simulink model "Model_Simulation"  (R2016a)
settings: Solver=FixedStepAuto  StartTime=0.0  StopTime=5  FixedStep=2e-6  RelTol=1e-3
values from neighbouring files (symbols this model uses):
  C = 3060e-6    (= 0.00306)    [Controle_Inversor_UR_D.m]
  Ki_i_disc = wc*Rf    (= 44.2477838534)    [Controle_Inversor_UR_D.m]
  Ki_i_disc_b = wc_b*Rb/Vdc    (= 0.0983284085631)    [Controle_Inversor_UR_D.m]
  Ki_q_disc = wq/H    [Controle_Inversor_UR_D.m]
  Ki_v_disc_b = wc_bv/Req    (= 14.5799013102)    [Controle_Inversor_UR_D.m]
  Ki_vdc_disc = ((wvdc)^2*C)/Gt    [Controle_Inversor_UR_D.m]
  Kp_i_disc = wc*Lf    (= 2.19688771906)    [Controle_Inversor_UR_D.m]
  Kp_i_disc_b = wc_b*Lb/Vdc    (= 0.00545604673435)    [Controle_Inversor_UR_D.m]
  Kp_q_disc = Ki_q_disc*(Lf/Kp_i_disc)    [Controle_Inversor_UR_D.m]
  Kp_v_disc_b = wc_bv*Cin    (= 0.0356301510224)    [Controle_Inversor_UR_D.m]
  Kp_vdc_disc = (2*ksi_vdc*wvdc*C)/Gt    [Controle_Inversor_UR_D.m]
  Lf = (0.0012+2.8949e-04)    (= 0.00148949)    [Controle_Inversor_UR_D.m]
  Tsw = 1/fsw    (= 0.0002)    [Controle_Inversor_UR_D.m]
  w = 2*pi*60    (= 376.991118431)    [Controle_Inversor_UR_D.m]
undefined symbols (not defined in the file or in its folder): D1, dEgdT, Delta, EgRef, gcbh, k1, Rsh_array5pc, sigbuilder_block, sps_rtmsupport, Tref_K, VT_ref
libraries: powerlib x179, simulink x14, powerlib_meascontrol x13, spsPVarrayModel x12
(part 1 of 20)
settings Model: Creator=lucca  LastModifiedBy=lucca

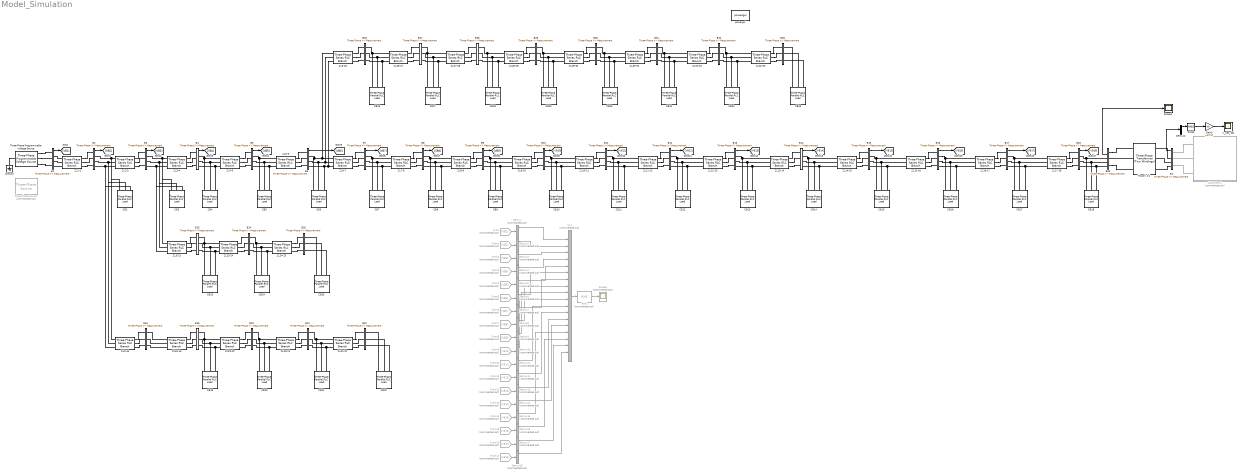
== system Model_Simulation ==
  B1 : powerlib/Measurements/Three-Phase V-I Measurement  VoltageMeasurement=phase-to-ground  SetLabelV=off  LabelV=Vabc  Vpu=off  VpuLL=off  CurrentMeasurement=yes  SetLabelI=off  LabelI=Iabc  Ipu=off  Pbase=100e6  Vbase=1.06  OutputType=Complex  PhasorSimulation=off  PSBequivalent=0
  "B1 " : powerlib/Measurements/Three-Phase V-I Measurement  VoltageMeasurement=phase-to-phase  SetLabelV=off  LabelV=Vabc  Vpu=off  VpuLL=off  CurrentMeasurement=no  SetLabelI=off  LabelI=Iabc  Ipu=off  Pbase=100e6  Vbase=1.06  OutputType=Complex  PhasorSimulation=off  PSBequivalent=0
  B{2..18} (17 alike) : powerlib/Measurements/Three-Phase V-I Measurement  VoltageMeasurement=phase-to-phase  SetLabelV=off  LabelV=Vabc  Vpu=off  VpuLL=off  CurrentMeasurement=no  SetLabelI=off  LabelI=Iabc  Ipu=off  Pbase=100e6  Vbase=1.06  OutputType=Complex  PhasorSimulation=off  PSBequivalent=0
  B{19..34} (16 alike) : powerlib/Measurements/Three-Phase V-I Measurement  VoltageMeasurement=no  SetLabelV=off  LabelV=Vabc  Vpu=off  VpuLL=off  CurrentMeasurement=no  SetLabelI=off  LabelI=Iabc  Ipu=off  Pbase=100e6  Vbase=1.06  OutputType=Complex  PhasorSimulation=off  PSBequivalent=0
  B35 : powerlib/Measurements/Three-Phase V-I Measurement  VoltageMeasurement=phase-to-ground  SetLabelV=off  LabelV=Vabc  Vpu=off  VpuLL=off  CurrentMeasurement=yes  SetLabelI=off  LabelI=Iabc  Ipu=off  Pbase=100e6  Vbase=1.06  OutputType=Complex  PhasorSimulation=off  PSBequivalent=0
  CB{6,9..10,16..17,28} (6 alike) : powerlib/Elements/Three-Phase Parallel RLC Load  LConnTagsString=A|B|C  Configuration=Y (grounded)  NominalVoltage=13.8e3  Vabc=[1e3 1e3 1e3]  Vabcp=[1e3 1e3 1e3]  NominalFrequency=60  UnbalancedPower=off  ActivePower=0.06e6  InductivePower=0.02e6  CapacitivePower=0  Pabc=[10e3 9e3 11e3]  QLabc=[100 90 110]  QCabc=[100 90 110]  Pabcp=[10e3 9e3 11e3]  QLabcp=[100 90 110]  QCabcp=[100 90 110]  Measurements=None  LoadType=constant Z
  CB11 : powerlib/Elements/Three-Phase Parallel RLC Load  LConnTagsString=A|B|C  Configuration=Y (grounded)  NominalVoltage=13.8e3  Vabc=[1e3 1e3 1e3]  Vabcp=[1e3 1e3 1e3]  NominalFrequency=60  UnbalancedPower=off  ActivePower=0.045e6  InductivePower=0.03e6  CapacitivePower=0  Pabc=[10e3 9e3 11e3]  QLabc=[100 90 110]  QCabc=[100 90 110]  Pabcp=[10e3 9e3 11e3]  QLabcp=[100 90 110]  QCabcp=[100 90 110]  Measurements=None  LoadType=constant Z
  CB12 : powerlib/Elements/Three-Phase Parallel RLC Load  LConnTagsString=A|B|C  Configuration=Y (grounded)  NominalVoltage=13.8e3  Vabc=[1e3 1e3 1e3]  Vabcp=[1e3 1e3 1e3]  NominalFrequency=60  UnbalancedPower=off  ActivePower=0.06e6  InductivePower=0.035e6  CapacitivePower=0  Pabc=[10e3 9e3 11e3]  QLabc=[100 90 110]  QCabc=[100 90 110]  Pabcp=[10e3 9e3 11e3]  QLabcp=[100 90 110]  QCabcp=[100 90 110]  Measurements=None  LoadType=constant Z
  CB13 : powerlib/Elements/Three-Phase Parallel RLC Load  LConnTagsString=A|B|C  Configuration=Y (grounded)  NominalVoltage=13.8e3  Vabc=[1e3 1e3 1e3]  Vabcp=[1e3 1e3 1e3]  NominalFrequency=60  UnbalancedPower=off  ActivePower=0.06e6  InductivePower=0.035e6  CapacitivePower=0  Pabc=[10e3 9e3 11e3]  QLabc=[100 90 110]  QCabc=[100 90 110]  Pabcp=[10e3 9e3 11e3]  QLabcp=[100 90 110]  QCabcp=[100 90 110]  Measurements=None  LoadType=constant Z
  CB14 : powerlib/Elements/Three-Phase Parallel RLC Load  LConnTagsString=A|B|C  Configuration=Y (grounded)  NominalVoltage=13.8e3  Vabc=[1e3 1e3 1e3]  Vabcp=[1e3 1e3 1e3]  NominalFrequency=60  UnbalancedPower=off  ActivePower=0.12e6  InductivePower=0.08e6  CapacitivePower=0  Pabc=[10e3 9e3 11e3]  QLabc=[100 90 110]  QCabc=[100 90 110]  Pabcp=[10e3 9e3 11e3]  QLabcp=[100 90 110]  QCabcp=[100 90 110]  Measurements=None  LoadType=constant Z
  CB15 : powerlib/Elements/Three-Phase Parallel RLC Load  LConnTagsString=A|B|C  Configuration=Y (grounded)  NominalVoltage=13.8e3  Vabc=[1e3 1e3 1e3]  Vabcp=[1e3 1e3 1e3]  NominalFrequency=60  UnbalancedPower=off  ActivePower=0.06e6  InductivePower=0.01e6  CapacitivePower=0  Pabc=[10e3 9e3 11e3]  QLabc=[100 90 110]  QCabc=[100 90 110]  Pabcp=[10e3 9e3 11e3]  QLabcp=[100 90 110]  QCabcp=[100 90 110]  Measurements=None  LoadType=constant Z
  CB{3,18..22} (6 alike) : powerlib/Elements/Three-Phase Parallel RLC Load  LConnTagsString=A|B|C  Configuration=Y (grounded)  NominalVoltage=13.8e3  Vabc=[1e3 1e3 1e3]  Vabcp=[1e3 1e3 1e3]  NominalFrequency=60  UnbalancedPower=off  ActivePower=0.09e6  InductivePower=0.04e6  CapacitivePower=0  Pabc=[10e3 9e3 11e3]  QLabc=[100 90 110]  QCabc=[100 90 110]  Pabcp=[10e3 9e3 11e3]  QLabcp=[100 90 110]  QCabcp=[100 90 110]  Measurements=None  LoadType=constant Z
  CB2 : powerlib/Elements/Three-Phase Parallel RLC Load  LConnTagsString=A|B|C  Configuration=Y (grounded)  NominalVoltage=13.8e3  Vabc=[1e3 1e3 1e3]  Vabcp=[1e3 1e3 1e3]  NominalFrequency=60  UnbalancedPower=off  ActivePower=0.1e6  InductivePower=0.06e6  CapacitivePower=0  Pabc=[10e3 9e3 11e3]  QLabc=[100 90 110]  QCabc=[100 90 110]  Pabcp=[10e3 9e3 11e3]  QLabcp=[100 90 110]  QCabcp=[100 90 110]  Measurements=None  LoadType=constant Z
  CB23 : powerlib/Elements/Three-Phase Parallel RLC Load  LConnTagsString=A|B|C  Configuration=Y (grounded)  NominalVoltage=13.8e3  Vabc=[1e3 1e3 1e3]  Vabcp=[1e3 1e3 1e3]  NominalFrequency=60  UnbalancedPower=off  ActivePower=0.09e6  InductivePower=0.05e6  CapacitivePower=0  Pabc=[10e3 9e3 11e3]  QLabc=[100 90 110]  QCabc=[100 90 110]  Pabcp=[10e3 9e3 11e3]  QLabcp=[100 90 110]  QCabcp=[100 90 110]  Measurements=None  LoadType=constant Z
  CB24 : powerlib/Elements/Three-Phase Parallel RLC Load  LConnTagsString=A|B|C  Configuration=Y (grounded)  NominalVoltage=13.8e3  Vabc=[1e3 1e3 1e3]  Vabcp=[1e3 1e3 1e3]  NominalFrequency=60  UnbalancedPower=off  ActivePower=0.42e6  InductivePower=0.2e6  CapacitivePower=0  Pabc=[10e3 9e3 11e3]  QLabc=[100 90 110]  QCabc=[100 90 110]  Pabcp=[10e3 9e3 11e3]  QLabcp=[100 90 110]  QCabcp=[100 90 110]  Measurements=None  LoadType=constant Z
  CB25 : powerlib/Elements/Three-Phase Parallel RLC Load  LConnTagsString=A|B|C  Configuration=Y (grounded)  NominalVoltage=13.8e3  Vabc=[1e3 1e3 1e3]  Vabcp=[1e3 1e3 1e3]  NominalFrequency=60  UnbalancedPower=off  ActivePower=0.42e6  InductivePower=0.2e6  CapacitivePower=0  Pabc=[10e3 9e3 11e3]  QLabc=[100 90 110]  QCabc=[100 90 110]  Pabcp=[10e3 9e3 11e3]  QLabcp=[100 90 110]  QCabcp=[100 90 110]  Measurements=None  LoadType=constant Z
  CB26 : powerlib/Elements/Three-Phase Parallel RLC Load  LConnTagsString=A|B|C  Configuration=Y (grounded)  NominalVoltage=13.8e3  Vabc=[1e3 1e3 1e3]  Vabcp=[1e3 1e3 1e3]  NominalFrequency=60  UnbalancedPower=off  ActivePower=0.06e6  InductivePower=0.025e6  CapacitivePower=0  Pabc=[10e3 9e3 11e3]  QLabc=[100 90 110]  QCabc=[100 90 110]  Pabcp=[10e3 9e3 11e3]  QLabcp=[100 90 110]  QCabcp=[100 90 110]  Measurements=None  LoadType=constant Z
  CB27 : powerlib/Elements/Three-Phase Parallel RLC Load  LConnTagsString=A|B|C  Configuration=Y (grounded)  NominalVoltage=13.8e3  Vabc=[1e3 1e3 1e3]  Vabcp=[1e3 1e3 1e3]  NominalFrequency=60  UnbalancedPower=off  ActivePower=0.06e6  InductivePower=0.025e6  CapacitivePower=0  Pabc=[10e3 9e3 11e3]  QLabc=[100 90 110]  QCabc=[100 90 110]  Pabcp=[10e3 9e3 11e3]  QLabcp=[100 90 110]  QCabcp=[100 90 110]  Measurements=None  LoadType=constant Z
  CB29 : powerlib/Elements/Three-Phase Parallel RLC Load  LConnTagsString=A|B|C  Configuration=Y (grounded)  NominalVoltage=13.8e3  Vabc=[1e3 1e3 1e3]  Vabcp=[1e3 1e3 1e3]  NominalFrequency=60  UnbalancedPower=off  ActivePower=0.12e6  InductivePower=0.07e6  CapacitivePower=0  Pabc=[10e3 9e3 11e3]  QLabc=[100 90 110]  QCabc=[100 90 110]  Pabcp=[10e3 9e3 11e3]  QLabcp=[100 90 110]  QCabcp=[100 90 110]  Measurements=None  LoadType=constant Z
  CB30 : powerlib/Elements/Three-Phase Parallel RLC Load  LConnTagsString=A|B|C  Configuration=Y (grounded)  NominalVoltage=13.8e3  Vabc=[1e3 1e3 1e3]  Vabcp=[1e3 1e3 1e3]  NominalFrequency=60  UnbalancedPower=off  ActivePower=0.2e6  InductivePower=0.1e6  CapacitivePower=0  Pabc=[10e3 9e3 11e3]  QLabc=[100 90 110]  QCabc=[100 90 110]  Pabcp=[10e3 9e3 11e3]  QLabcp=[100 90 110]  QCabcp=[100 90 110]  Measurements=None  LoadType=constant Z
  CB31 : powerlib/Elements/Three-Phase Parallel RLC Load  LConnTagsString=A|B|C  Configuration=Y (grounded)  NominalVoltage=13.8e3  Vabc=[1e3 1e3 1e3]  Vabcp=[1e3 1e3 1e3]  NominalFrequency=60  UnbalancedPower=off  ActivePower=0.15e6  InductivePower=0.07e6  CapacitivePower=0  Pabc=[10e3 9e3 11e3]  QLabc=[100 90 110]  QCabc=[100 90 110]  Pabcp=[10e3 9e3 11e3]  QLabcp=[100 90 110]  QCabcp=[100 90 110]  Measurements=None  LoadType=constant Z
  CB32 : powerlib/Elements/Three-Phase Parallel RLC Load  LConnTagsString=A|B|C  Configuration=Y (grounded)  NominalVoltage=13.8e3  Vabc=[1e3 1e3 1e3]  Vabcp=[1e3 1e3 1e3]  NominalFrequency=60  UnbalancedPower=off  ActivePower=0.21e6  InductivePower=0.1e6  CapacitivePower=0  Pabc=[10e3 9e3 11e3]  QLabc=[100 90 110]  QCabc=[100 90 110]  Pabcp=[10e3 9e3 11e3]  QLabcp=[100 90 110]  QCabcp=[100 90 110]  Measurements=None  LoadType=constant Z
  CB33 : powerlib/Elements/Three-Phase Parallel RLC Load  LConnTagsString=A|B|C  Configuration=Y (grounded)  NominalVoltage=13.8e3  Vabc=[1e3 1e3 1e3]  Vabcp=[1e3 1e3 1e3]  NominalFrequency=60  UnbalancedPower=off  ActivePower=0.06e6  InductivePower=0.04e6  CapacitivePower=0  Pabc=[10e3 9e3 11e3]  QLabc=[100 90 110]  QCabc=[100 90 110]  Pabcp=[10e3 9e3 11e3]  QLabcp=[100 90 110]  QCabcp=[100 90 110]  Measurements=None  LoadType=constant Z
  CB4 : powerlib/Elements/Three-Phase Parallel RLC Load  LConnTagsString=A|B|C  Configuration=Y (grounded)  NominalVoltage=13.8e3  Vabc=[1e3 1e3 1e3]  Vabcp=[1e3 1e3 1e3]  NominalFrequency=60  UnbalancedPower=off  ActivePower=0.12e6  InductivePower=0.08e6  CapacitivePower=0  Pabc=[10e3 9e3 11e3]  QLabc=[100 90 110]  QCabc=[100 90 110]  Pabcp=[10e3 9e3 11e3]  QLabcp=[100 90 110]  QCabcp=[100 90 110]  Measurements=None  LoadType=constant Z
  CB5 : powerlib/Elements/Three-Phase Parallel RLC Load  LConnTagsString=A|B|C  Configuration=Y (grounded)  NominalVoltage=13.8e3  Vabc=[1e3 1e3 1e3]  Vabcp=[1e3 1e3 1e3]  NominalFrequency=60  UnbalancedPower=off  ActivePower=0.06e6  InductivePower=0.03e6  CapacitivePower=0  Pabc=[10e3 9e3 11e3]  QLabc=[100 90 110]  QCabc=[100 90 110]  Pabcp=[10e3 9e3 11e3]  QLabcp=[100 90 110]  QCabcp=[100 90 110]  Measurements=None  LoadType=constant Z
  CB7 : powerlib/Elements/Three-Phase Parallel RLC Load  LConnTagsString=A|B|C  Configuration=Y (grounded)  NominalVoltage=13.8e3  Vabc=[1e3 1e3 1e3]  Vabcp=[1e3 1e3 1e3]  NominalFrequency=60  UnbalancedPower=off  ActivePower=0.2e6  InductivePower=0.1e6  CapacitivePower=0  Pabc=[10e3 9e3 11e3]  QLabc=[100 90 110]  QCabc=[100 90 110]  Pabcp=[10e3 9e3 11e3]  QLabcp=[100 90 110]  QCabcp=[100 90 110]  Measurements=None  LoadType=constant Z
  CB8 : powerlib/Elements/Three-Phase Parallel RLC Load  LConnTagsString=A|B|C  Configuration=Y (grounded)  NominalVoltage=13.8e3  Vabc=[1e3 1e3 1e3]  Vabcp=[1e3 1e3 1e3]  NominalFrequency=60  UnbalancedPower=off  ActivePower=0.2e6  InductivePower=0.1e6  CapacitivePower=0  Pabc=[10e3 9e3 11e3]  QLabc=[100 90 110]  QCabc=[100 90 110]  Pabcp=[10e3 9e3 11e3]  QLabcp=[100 90 110]  QCabcp=[100 90 110]  Measurements=None  LoadType=constant Z
  Demux{,1,3..18} (18 alike) : Demux  Commented=on  Outputs=3
  Demux2 : Demux  Outputs=3
  From : From  Commented=on  GotoTag=VB1
  From1 : From  Commented=on  GotoTag=VB2
  From10 : From  Commented=on  GotoTag=VB11
  From11 : From  Commented=on  GotoTag=VB12
  From12 : From  Commented=on  GotoTag=VB13
  From13 : From  Commented=on  GotoTag=VB14
  From14 : From  Commented=on  GotoTag=VB15
  From15 : From  Commented=on  GotoTag=VB16
  From16 : From  Commented=on  GotoTag=VB17
  From17 : From  Commented=on  GotoTag=VB18
  From2 : From  Commented=on  GotoTag=VB3
  From3 : From  Commented=on  GotoTag=VB4
  From4 : From  Commented=on  GotoTag=VB5
  From5 : From  Commented=on  GotoTag=VB6
  From6 : From  Commented=on  GotoTag=VB7
  From7 : From  Commented=on  GotoTag=VB8
  From8 : From  Commented=on  GotoTag=VB9
  From9 : From  Commented=on  GotoTag=VB10
  Gain3 : Gain  Gain=sqrt(2)
  Ground : powerlib/Elements/Ground  LConnTagsString=a
  Mux : Mux  Commented=on  Inputs=18
  RMS : powerlib_meascontrol/Measurements/RMS  Commented=on  TrueRMS=on  Freq=60  RMSInit=13800  Ts=0
  RMS5 : powerlib_meascontrol/Measurements/RMS  TrueRMS=on  Freq=60  RMSInit=120  Ts=0
  Scope2 : Scope
  Scope3 : Scope  Commented=on
  Subsystem2 : Subsystem  Commented=on
  Three-Phase Programmable Voltage Source : powerlib/Electrical Sources/Three-Phase Programmable Voltage Source  PositiveSequence=[13.8e3 0 60]  VariationEntity=Amplitude  VariationType=Table of time-amplitude pairs  VariationTypeAlt=Step  VariationStep=0.5  VariationRate=10  VariationMagnitude=0.3  VariationFrequency=2  VariationTiming=[1 2]  VariationPhaseA=off  Amplitudes=[1 0.7 1]  TimeValues=[0 2 3]  HarmonicGeneration=off  HarmonicA=[3 0.2 -25 0]  HarmonicB=[2 0.15 35 2]  Timing="[0.05  3]"  BusType=swing  Pref=0  Qref=0  Qmin=-inf  Qmax=inf
  Three-Phase Source : powerlib/Electrical Sources/Three-Phase Source  Commented=on  InternalConnection=Yg  VoltagePhases=off  Voltage=13.8e3  PhaseAngle=0  Voltage_phases=[25e3 25e3 25e3]/sqrt(3)  PhaseAngles_phases=[0 -120 +120]  Frequency=60  NonIdealSource=off  SpecifyImpedance=off  Resistance=0.8929  Inductance=16.58e-3  ShortCircuitLevel=100e6  BaseVoltage=25e3  XRratio=7  BusType=swing  Pref=10e3  Qref=0  Prefabc=[10e3, 10e3, 10e3]  Qrefabc=[0, 0, 0]  Qmin=-inf  Qmax=inf
  Transf. 4-1 : powerlib/Elements/Three-Phase Transformer (Two Windings)  Winding1Connection=Delta (D1)  Winding2Connection=Yg  CoreType=Three single-phase transformers  SetSaturation=off  Hysteresis=off  DataFile='hysteresis'  SetInitialFlux=off  Measurements=None  UNITS=pu  NominalPower=[ 300e3 , 60 ]  Winding1=[13800 0 0.05/2]  Winding2=[800 0 0.05/2]  Rm=370.3704  Lm=14.4834  L0=0.49999  Saturation=[0 0;0.006 1.2;2.4999 1.52]  InitialFluxes=[0.80003 -0.80003 0.70001]  MoreParameters=off  BreakLoop=off  DataType=off  TransfoNumber=1
  V_sec_GD : Scope
  ZL1-2 : powerlib/Elements/Three-Phase Series RLC Branch  LConnTagsString=A|B|C  RConnTagsString=A|B|C  BranchType=RL  Resistance=0.057525912  Inductance=7.7784e-05  Capacitance=1e-6  Measurements=None
  ZL10-11 : powerlib/Elements/Three-Phase Series RLC Branch  LConnTagsString=A|B|C  RConnTagsString=A|B|C  BranchType=RL  Resistance=0.122663712  Inductance=1.0758e-04  Capacitance=1e-6  Measurements=None
  ZL11-12 : powerlib/Elements/Three-Phase Series RLC Branch  LConnTagsString=A|B|C  RConnTagsString=A|B|C  BranchType=RL  Resistance=0.233597628  Inductance=2.0489e-04  Capacitance=1e-6  Measurements=None
  ZL12-13 : powerlib/Elements/Three-Phase Series RLC Branch  LConnTagsString=A|B|C  RConnTagsString=A|B|C  BranchType=RL  Resistance=0.915922324  Inductance=0.0019  Capacitance=1e-6  Measurements=None
  ZL13-14 : powerlib/Elements/Three-Phase Series RLC Branch  LConnTagsString=A|B|C  RConnTagsString=A|B|C  BranchType=RL  Resistance=0.337917936  Inductance=0.0012  Capacitance=1e-6  Measurements=None
  ZL14-15 : powerlib/Elements/Three-Phase Series RLC Branch  LConnTagsString=A|B|C  RConnTagsString=A|B|C  BranchType=RL  Resistance=0.368739846  Inductance=8.7054e-04  Capacitance=1e-6  Measurements=None
  ZL15-16 : powerlib/Elements/Three-Phase Series RLC Branch  LConnTagsString=A|B|C  RConnTagsString=A|B|C  BranchType=RL  Resistance=0.465635443  Inductance=9.0198e-04  Capacitance=1e-6  Measurements=None
  ZL16-17 : powerlib/Elements/Three-Phase Series RLC Branch  LConnTagsString=A|B|C  RConnTagsString=A|B|C  BranchType=RL  Resistance=0.804239697  Inductance=0.0028  Capacitance=1e-6  Measurements=None
  ZL17-18 : powerlib/Elements/Three-Phase Series RLC Branch  LConnTagsString=A|B|C  RConnTagsString=A|B|C  BranchType=RL  Resistance=0.456713311  Inductance=9.4998e-04  Capacitance=1e-6  Measurements=None
  ZL19-20 : powerlib/Elements/Three-Phase Series RLC Branch  LConnTagsString=A|B|C  RConnTagsString=A|B|C  BranchType=RL  Resistance=0.938508419  Inductance=0.0022  Capacitance=1e-6  Measurements=None
  ZL2-3 : powerlib/Elements/Three-Phase Series RLC Branch  LConnTagsString=A|B|C  RConnTagsString=A|B|C  BranchType=RL  Resistance=0.307595167  Inductance=4.1557e-04  Capacitance=1e-6  Measurements=None
  ZL2-34 : powerlib/Elements/Three-Phase Series RLC Branch  LConnTagsString=A|B|C  RConnTagsString=A|B|C  BranchType=RL  Resistance=0.057525912  Inductance=7.7784e-05  Capacitance=1e-6  Measurements=None
  ZL20-21 : powerlib/Elements/Three-Phase Series RLC Branch  LConnTagsString=A|B|C  RConnTagsString=A|B|C  BranchType=RL  Resistance=0.255497406  Inductance=7.9176e-04  Capacitance=1e-6  Measurements=None
  ZL21-22 : powerlib/Elements/Three-Phase Series RLC Branch  LConnTagsString=A|B|C  RConnTagsString=A|B|C  BranchType=RL  Resistance=0.442300637  Inductance=0.0016  Capacitance=1e-6  Measurements=None
  ZL23-24 : powerlib/Elements/Three-Phase Series RLC Branch  LConnTagsString=A|B|C  RConnTagsString=A|B|C  BranchType=RL  Resistance=0.560284909  Inductance=0.0012  Capacitance=1e-6  Measurements=None
  ZL24-25 : powerlib/Elements/Three-Phase Series RLC Branch  LConnTagsString=A|B|C  RConnTagsString=A|B|C  BranchType=RL  Resistance=0.559037059  Inductance=0.0012  Capacitance=1e-6  Measurements=None
  ZL26-27 : powerlib/Elements/Three-Phase Series RLC Branch  LConnTagsString=A|B|C  RConnTagsString=A|B|C  BranchType=RL  Resistance=0.177319567  Inductance=2.3948e-04  Capacitance=1e-6  Measurements=None
  ZL27-28 : powerlib/Elements/Three-Phase Series RLC Branch  LConnTagsString=A|B|C  RConnTagsString=A|B|C  BranchType=RL  Resistance=0.660736881  Inductance=0.0015  Capacitance=1e-6  Measurements=None
  ZL28-29 : powerlib/Elements/Three-Phase Series RLC Branch  LConnTagsString=A|B|C  RConnTagsString=A|B|C  BranchType=RL  Resistance=0.501760717  Inductance=0.0012  Capacitance=1e-6  Measurements=None
  ZL29-30 : powerlib/Elements/Three-Phase Series RLC Branch  LConnTagsString=A|B|C  RConnTagsString=A|B|C  BranchType=RL  Resistance=0.316642084  Inductance=4.2782e-04  Capacitance=1e-6  Measurements=None
  ZL3-23 : powerlib/Elements/Three-Phase Series RLC Branch  LConnTagsString=A|B|C  RConnTagsString=A|B|C  BranchType=RL  Resistance=0.28151509  Inductance=5.1024e-04  Capacitance=1e-6  Measurements=None
  ZL3-4 : powerlib/Elements/Three-Phase Series RLC Branch  LConnTagsString=A|B|C  RConnTagsString=A|B|C  BranchType=RL  Resistance=0.228356656  Inductance=3.0850e-04  Capacitance=1e-6  Measurements=None
  ZL30-31 : powerlib/Elements/Three-Phase Series RLC Branch  LConnTagsString=A|B|C  RConnTagsString=A|B|C  BranchType=RL  Resistance=0.607952801  Inductance=0.0016  Capacitance=1e-6  Measurements=None
  ZL31-32 : powerlib/Elements/Three-Phase Series RLC Branch  LConnTagsString=A|B|C  RConnTagsString=A|B|C  BranchType=RL  Resistance=0.193728802  Inductance=5.9895e-04  Capacitance=1e-6  Measurements=None
  ZL32-33 : powerlib/Elements/Three-Phase Series RLC Branch  LConnTagsString=A|B|C  RConnTagsString=A|B|C  BranchType=RL  Resistance=0.212758523  Inductance=8.7749e-04  Capacitance=1e-6  Measurements=None
  ZL34-19 : powerlib/Elements/Three-Phase Series RLC Branch  LConnTagsString=A|B|C  RConnTagsString=A|B|C  BranchType=RL  Resistance=0.938508419  Inductance=0.0022  Capacitance=1e-6  Measurements=None
  ZL4-5 : powerlib/Elements/Three-Phase Series RLC Branch  LConnTagsString=A|B|C  RConnTagsString=A|B|C  BranchType=RL  Resistance=0.237777928  Inductance=3.2124e-04  Capacitance=1e-6  Measurements=None
  ZL5-6 : powerlib/Elements/Three-Phase Series RLC Branch  LConnTagsString=A|B|C  RConnTagsString=A|B|C  BranchType=RL  Resistance=0.510994811  Inductance=0.0012  Capacitance=1e-6  Measurements=None
  ZL6-26 : powerlib/Elements/Three-Phase Series RLC Branch  LConnTagsString=A|B|C  RConnTagsString=A|B|C  BranchType=RL  Resistance=0.126656834  Inductance=1.7113e-04  Capacitance=1e-6  Measurements=None
  ZL6-7 : powerlib/Elements/Three-Phase Series RLC Branch  LConnTagsString=A|B|C  RConnTagsString=A|B|C  BranchType=RL  Resistance=0.116798814  Inductance=0.0010  Capacitance=1e-6  Measurements=None
  ZL7-8 : powerlib/Elements/Three-Phase Series RLC Branch  LConnTagsString=A|B|C  RConnTagsString=A|B|C  BranchType=RL  Resistance=0.44386045  Inductance=3.8909e-04  Capacitance=1e-6  Measurements=None
  ZL8-9 : powerlib/Elements/Three-Phase Series RLC Branch  LConnTagsString=A|B|C  RConnTagsString=A|B|C  BranchType=RL  Resistance=0.642643047  Inductance=0.0012  Capacitance=1e-6  Measurements=None
  ZL9-10 : powerlib/Elements/Three-Phase Series RLC Branch  LConnTagsString=A|B|C  RConnTagsString=A|B|C  BranchType=RL  Resistance=0.651378001  Inductance=0.0012  Capacitance=1e-6  Measurements=None
  powergui : powerlib/powergui  Priority=1  SimulationMode=Discrete  SolverType=Tustin  SampleTime=2e-6  frequency=60  SPID=off  DisableSnubberDevices=off  DisableRonSwitches=off  DisableVfSwitches=off  SwTol=0  DisplayEquations=off  Interpol=off  ExternalGateDelay=off  methode=off  Ts=10  FunctionMessages=off  echomessages=off  HookPort=off  EnableUseOfTLC=off  x0status=blocks  frequencyindice=60  Pbase=100e6  ErrMax=0.0001  Iterations=50  UnitsV=kV  UnitsW=MW  buscounter=0  RestoreLinks=warning  ResistiveCurrentMeasurement=off  Frange=[0:2:500]  Ylog=off  Xlog=on  ShowGrid=off  save=off  variable=ZData  structure=0  ZoomFFT=off  StartTime=0.0  cycles=1  DisplayStyle=1  fundamental=60  FreqAxis=off  MaxFrequency=1000  frequencyindicesteady=1  RmsSteady=1  display=off
  wires:
  B1/1 -> Demux2/1
  RMS5/1 -> Gain3/1
  Gain3/1 -> V_sec_GD/1
  Demux2/1 -> RMS5/1
  "B1 "/1 -> [VB1]
  B2/1 -> [VB2]
  B3/1 -> [VB3]
  B4/1 -> [VB4]
  B5/1 -> [VB5]
  B6/1 -> [VB6]
  B7/1 -> [VB7]
  B8/1 -> [VB8]
  B9/1 -> [VB9]
  B10/1 -> [VB10]
  B11/1 -> [VB11]
  B12/1 -> [VB12]
  B13/1 -> [VB13]
  B14/1 -> [VB14]
  B15/1 -> [VB15]
  B16/1 -> [VB16]
  B17/1 -> [VB17]
  B18/1 -> [VB18]
  Mux/1 -> RMS/1
  Demux/1 -> Mux/1
  Demux1/1 -> Mux/2
  Demux3/1 -> Mux/3
  Demux4/1 -> Mux/4
  Demux5/1 -> Mux/5
  Demux6/1 -> Mux/6
  Demux7/1 -> Mux/7
  Demux8/1 -> Mux/8
  Demux9/1 -> Mux/9
  Demux10/1 -> Mux/10
  Demux11/1 -> Mux/11
  Demux12/1 -> Mux/12
  Demux13/1 -> Mux/13
  Demux14/1 -> Mux/14
  Demux15/1 -> Mux/15
  Demux16/1 -> Mux/16
  Demux17/1 -> Mux/17
  Demux18/1 -> Mux/18
  From/1 -> Demux/1
  From1/1 -> Demux1/1
  From2/1 -> Demux3/1
  From3/1 -> Demux4/1
  From4/1 -> Demux5/1
  From5/1 -> Demux6/1
  From6/1 -> Demux7/1
  From7/1 -> Demux8/1
  From8/1 -> Demux9/1
  From9/1 -> Demux10/1
  From10/1 -> Demux11/1
  From11/1 -> Demux12/1
  From12/1 -> Demux13/1
  From13/1 -> Demux14/1
  From14/1 -> Demux15/1
  From15/1 -> Demux16/1
  From16/1 -> Demux17/1
  From17/1 -> Demux18/1
  RMS/1 -> Scope3/1
  B35/2 -> Scope2/1
  connections:
  ZL1-2/LConn1 -- "B1 "/RConn1
  ZL1-2/LConn2 -- "B1 "/RConn2
  ZL1-2/LConn3 -- "B1 "/RConn3
  ZL1-2/RConn2 -- B2/LConn2
  ZL1-2/RConn1 -- B2/LConn1
  ZL1-2/RConn3 -- B2/LConn3
  ZL2-3/LConn1 -- ZL2-34/LConn1 -- CB2/LConn1 -- B2/RConn1
  ZL2-3/LConn2 -- ZL2-34/LConn2 -- CB2/LConn2 -- B2/RConn2
  ZL2-3/LConn3 -- CB2/LConn3 -- ZL2-34/LConn3 -- B2/RConn3
  ZL2-3/RConn3 -- B3/LConn3
  ZL2-3/RConn2 -- B3/LConn2
  ZL2-3/RConn1 -- B3/LConn1
  ZL3-4/LConn1 -- CB3/LConn1 -- ZL3-23/LConn1 -- B3/RConn1
  ZL3-4/LConn2 -- CB3/LConn2 -- ZL3-23/LConn2 -- B3/RConn2
  ZL3-4/LConn3 -- CB3/LConn3 -- ZL3-23/LConn3 -- B3/RConn3
  ZL3-4/RConn3 -- B4/LConn3
  ZL3-4/RConn2 -- B4/LConn2
  ZL3-4/RConn1 -- B4/LConn1
  ZL4-5/LConn1 -- CB4/LConn1 -- B4/RConn1
  ZL4-5/LConn2 -- CB4/LConn2 -- B4/RConn2
  ZL4-5/LConn3 -- B4/RConn3 -- CB4/LConn3
  B5/LConn3 -- ZL4-5/RConn3
  ZL4-5/RConn2 -- B5/LConn2
  ZL4-5/RConn1 -- B5/LConn1
  ZL5-6/LConn3 -- CB5/LConn3 -- B5/RConn3
  ZL5-6/LConn1 -- CB5/LConn1 -- B5/RConn1
  ZL5-6/RConn2 -- B6/LConn2
  ZL5-6/RConn1 -- B6/LConn1
  ZL5-6/LConn2 -- CB5/LConn2 -- B5/RConn2
  ZL5-6/RConn3 -- B6/LConn3
  ZL6-7/RConn2 -- B7/LConn2
  ZL6-7/LConn2 -- ZL6-26/LConn2 -- CB6/LConn2 -- B6/RConn2
  ZL6-7/LConn1 -- ZL6-26/LConn1 -- CB6/LConn1 -- B6/RConn1
  ZL6-7/LConn3 -- ZL6-26/LConn3 -- CB6/LConn3 -- B6/RConn3
  ZL6-7/RConn1 -- B7/LConn1
  ZL6-7/RConn3 -- B7/LConn3
  ZL7-8/RConn1 -- B8/LConn1
  ZL7-8/RConn3 -- B8/LConn3
  ZL7-8/LConn3 -- CB7/LConn3 -- B7/RConn3
  ZL7-8/RConn2 -- B8/LConn2
  ZL7-8/LConn2 -- CB7/LConn2 -- B7/RConn2
  ZL7-8/LConn1 -- CB7/LConn1 -- B7/RConn1
  ZL8-9/RConn3 -- B9/LConn3
  ZL8-9/LConn3 -- CB8/LConn3 -- B8/RConn3
  ZL8-9/RConn1 -- B9/LConn1
  ZL8-9/LConn2 -- CB8/LConn2 -- B8/RConn2
  ZL8-9/LConn1 -- CB8/LConn1 -- B8/RConn1
  ZL8-9/RConn2 -- B9/LConn2
  ZL9-10/LConn2 -- CB9/LConn2 -- B9/RConn2
  ZL9-10/RConn1 -- B10/LConn1
  ZL9-10/LConn1 -- CB9/LConn1 -- B9/RConn1
  ZL9-10/LConn3 -- CB9/LConn3 -- B9/RConn3
  ZL9-10/RConn2 -- B10/LConn2
  ZL9-10/RConn3 -- B10/LConn3
  ZL10-11/LConn1 -- B10/RConn1 -- CB10/LConn1
  ZL10-11/RConn2 -- B11/LConn2
  ZL10-11/RConn1 -- B11/LConn1
  ZL10-11/LConn3 -- CB10/LConn3 -- B10/RConn3
  ZL10-11/RConn3 -- B11/LConn3
  ZL10-11/LConn2 -- CB10/LConn2 -- B10/RConn2
  ZL11-12/LConn2 -- CB11/LConn2 -- B11/RConn2
  ZL11-12/LConn3 -- CB11/LConn3 -- B11/RConn3
  ZL11-12/RConn2 -- B12/LConn2
  ZL11-12/RConn1 -- B12/LConn1
  ZL11-12/RConn3 -- B12/LConn3
  ZL11-12/LConn1 -- CB11/LConn1 -- B11/RConn1
  ZL12-13/LConn2 -- CB12/LConn2 -- B12/RConn2
  ZL12-13/LConn3 -- CB12/LConn3 -- B12/RConn3
  ZL12-13/RConn2 -- B13/LConn2
  ZL12-13/LConn1 -- CB12/LConn1 -- B12/RConn1
  ZL12-13/RConn3 -- B13/LConn3
  ZL12-13/RConn1 -- B13/LConn1
  ZL13-14/RConn3 -- B14/LConn3
  ZL13-14/LConn1 -- CB13/LConn1 -- B13/RConn1
  ZL13-14/RConn1 -- B14/LConn1
  ZL13-14/RConn2 -- B14/LConn2
  ZL13-14/LConn3 -- CB13/LConn3 -- B13/RConn3
  ZL13-14/LConn2 -- CB13/LConn2 -- B13/RConn2
  ZL14-15/LConn1 -- CB14/LConn1 -- B14/RConn1
  ZL14-15/LConn3 -- CB14/LConn3 -- B14/RConn3
  ZL14-15/RConn2 -- B15/LConn2
  ZL14-15/RConn1 -- B15/LConn1
  ZL14-15/LConn2 -- CB14/LConn2 -- B14/RConn2
  ZL14-15/RConn3 -- B15/LConn3
  ZL15-16/RConn1 -- B16/LConn1
  ZL15-16/LConn3 -- CB15/LConn3 -- B15/RConn3
  ZL15-16/LConn1 -- CB15/LConn1 -- B15/RConn1
  ZL15-16/RConn3 -- B16/LConn3
  ZL15-16/RConn2 -- B16/LConn2
  ZL15-16/LConn2 -- CB15/LConn2 -- B15/RConn2
  B16/RConn2 -- CB16/LConn2 -- ZL16-17/LConn2
  ZL16-17/RConn2 -- B17/LConn2
  B16/RConn3 -- CB16/LConn3 -- ZL16-17/LConn3
  ZL16-17/RConn1 -- B17/LConn1
  ZL16-17/RConn3 -- B17/LConn3
  B16/RConn1 -- CB16/LConn1 -- ZL16-17/LConn1
  ZL17-18/LConn2 -- B17/RConn2 -- CB17/LConn2
  ZL17-18/LConn1 -- CB17/LConn1 -- B17/RConn1
  ZL17-18/LConn3 -- B17/RConn3 -- CB17/LConn3
  ZL17-18/RConn3 -- B18/LConn3
  ZL17-18/RConn1 -- B18/LConn1
  ZL17-18/RConn2 -- B18/LConn2
  ZL34-19/RConn2 -- B19/LConn2
  ZL2-34/RConn3 -- B34/LConn3
  ZL19-20/LConn3 -- CB19/LConn3 -- B19/RConn3
  ZL34-19/LConn1 -- B34/RConn1
  ZL20-21/RConn2 -- B21/LConn2
  ZL20-21/LConn2 -- B20/RConn2 -- CB20/LConn2
  ZL20-21/LConn1 -- CB20/LConn1 -- B20/RConn1
  ZL20-21/LConn3 -- CB20/LConn3 -- B20/RConn3
  ZL20-21/RConn1 -- B21/LConn1
  ZL20-21/RConn3 -- B21/LConn3
  ZL34-19/RConn1 -- B19/LConn1
  ZL21-22/RConn1 -- B22/LConn1
  ZL21-22/RConn3 -- B22/LConn3
  ZL21-22/LConn3 -- CB21/LConn3 -- B21/RConn3
  ZL21-22/RConn2 -- B22/LConn2
  ZL21-22/LConn2 -- CB21/LConn2 -- B21/RConn2
  ZL21-22/LConn1 -- CB21/LConn1 -- B21/RConn1
  ZL34-19/LConn3 -- B34/RConn3
  ZL19-20/LConn1 -- CB19/LConn1 -- B19/RConn1
  ZL19-20/RConn2 -- B20/LConn2
  ZL19-20/RConn1 -- B20/LConn1
  ZL19-20/LConn2 -- CB19/LConn2 -- B19/RConn2
  B20/LConn3 -- ZL19-20/RConn3
  ZL34-19/LConn2 -- B34/RConn2
  ZL34-19/RConn3 -- B19/LConn3
  ZL2-34/RConn1 -- B34/LConn1
  ZL2-34/RConn2 -- B34/LConn2
  ZL23-24/RConn2 -- B24/LConn2
  ZL3-23/RConn3 -- B23/LConn3
  ZL24-25/LConn3 -- CB24/LConn3 -- B24/RConn3
  ZL23-24/LConn1 -- CB23/LConn1 -- B23/RConn1
  ZL23-24/RConn1 -- B24/LConn1
  ZL23-24/LConn3 -- CB23/LConn3 -- B23/RConn3
  ZL24-25/LConn1 -- CB24/LConn1 -- B24/RConn1
  ZL24-25/RConn2 -- B25/LConn2
  ZL24-25/RConn1 -- B25/LConn1
  ZL24-25/LConn2 -- B24/RConn2 -- CB24/LConn2
  B25/LConn3 -- ZL24-25/RConn3
  ZL23-24/LConn2 -- B23/RConn2 -- CB23/LConn2
  ZL23-24/RConn3 -- B24/LConn3
  ZL3-23/RConn1 -- B23/LConn1
  ZL3-23/RConn2 -- B23/LConn2
  ZL26-27/RConn2 -- B27/LConn2
  ZL26-27/LConn2 -- CB26/LConn2 -- B26/RConn2
  ZL26-27/LConn1 -- CB26/LConn1 -- B26/RConn1
  ZL26-27/LConn3 -- CB26/LConn3 -- B26/RConn3
  ZL26-27/RConn1 -- B27/LConn1
  ZL26-27/RConn3 -- B27/LConn3
  ZL32-33/LConn2 -- CB32/LConn2 -- B32/RConn2
  ZL32-33/LConn3 -- CB32/LConn3 -- B32/RConn3
  ZL32-33/RConn2 -- B33/LConn2
  ZL32-33/LConn1 -- CB32/LConn1 -- B32/RConn1
  ZL32-33/RConn3 -- B33/LConn3
  ZL32-33/RConn1 -- B33/LConn1
  ZL27-28/RConn1 -- B28/LConn1
  ZL27-28/RConn3 -- B28/LConn3
  ZL27-28/LConn3 -- CB27/LConn3 -- B27/RConn3
  ZL27-28/RConn2 -- B28/LConn2
  ZL27-28/LConn2 -- CB27/LConn2 -- B27/RConn2
  ZL27-28/LConn1 -- CB27/LConn1 -- B27/RConn1
  ZL30-31/LConn1 -- CB30/LConn1 -- B30/RConn1
  ZL30-31/RConn2 -- B31/LConn2
  ZL30-31/RConn1 -- B31/LConn1
  ZL30-31/LConn3 -- CB30/LConn3 -- B30/RConn3
  ZL30-31/RConn3 -- B31/LConn3
  ZL30-31/LConn2 -- CB30/LConn2 -- B30/RConn2
  ZL31-32/LConn2 -- B31/RConn2 -- CB31/LConn2
  ZL31-32/LConn3 -- CB31/LConn3 -- B31/RConn3
  ZL31-32/RConn2 -- B32/LConn2
  ZL31-32/RConn1 -- B32/LConn1
  ZL31-32/RConn3 -- B32/LConn3
  ZL31-32/LConn1 -- CB31/LConn1 -- B31/RConn1
  ZL6-26/RConn2 -- B26/LConn2
  ZL6-26/RConn1 -- B26/LConn1
  ZL28-29/RConn3 -- B29/LConn3
  ZL28-29/LConn3 -- CB28/LConn3 -- B28/RConn3
  ZL28-29/RConn1 -- B29/LConn1
  ZL28-29/LConn2 -- CB28/LConn2 -- B28/RConn2
  ZL28-29/LConn1 -- CB28/LConn1 -- B28/RConn1
  ZL28-29/RConn2 -- B29/LConn2
  B26/LConn3 -- ZL6-26/RConn3
  ZL29-30/LConn2 -- CB29/LConn2 -- B29/RConn2
  ZL29-30/RConn1 -- B30/LConn1
  ZL29-30/LConn1 -- CB29/LConn1 -- B29/RConn1
  ZL29-30/LConn3 -- CB29/LConn3 -- B29/RConn3
  ZL29-30/RConn2 -- B30/LConn2
  ZL29-30/RConn3 -- B30/LConn3
  CB18/LConn1 -- B18/RConn1 -- B35/RConn1
  CB18/LConn2 -- B35/RConn2 -- B18/RConn2
  CB18/LConn3 -- B35/RConn3 -- B18/RConn3
  CB22/LConn1 -- B22/RConn1
  CB22/LConn2 -- B22/RConn2
  CB22/LConn3 -- B22/RConn3
  CB25/LConn1 -- B25/RConn1
  CB25/LConn2 -- B25/RConn2
  CB25/LConn3 -- B25/RConn3
  CB33/LConn1 -- B33/RConn1
  CB33/LConn2 -- B33/RConn2
  CB33/LConn3 -- B33/RConn3
  Three-Phase Programmable Voltage Source/RConn2 -- "B1 "/LConn2
  Three-Phase Programmable Voltage Source/RConn1 -- "B1 "/LConn1
  Three-Phase Programmable Voltage Source/RConn3 -- "B1 "/LConn3
  Three-Phase Programmable Voltage Source/LConn1 -- Ground/LConn1
  B1/RConn1 -- Transf. 4-1/RConn1
  B1/RConn3 -- Transf. 4-1/RConn3
  B1/RConn2 -- Transf. 4-1/RConn2
  Transf. 4-1/LConn2 -- B35/LConn2
  B35/LConn1 -- Transf. 4-1/LConn1
  B35/LConn3 -- Transf. 4-1/LConn3
  Subsystem2/RConn1 -- B1/LConn1
  Subsystem2/RConn2 -- B1/LConn2
  Subsystem2/RConn3 -- B1/LConn3
